simulink model "plant_control"  (R2023a)
settings: Solver=VariableStepAuto  StartTime=0.0  StopTime=10.0  RelTol=1e-3
settings Model: Creator=timme  LastModifiedBy=timme

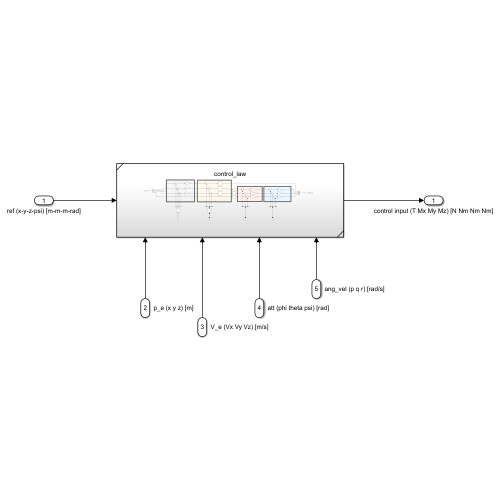
[thumbnail: Simulink's stored preview of the top-level diagram]
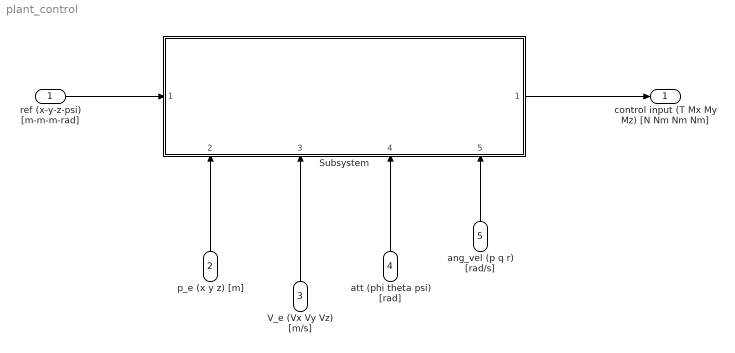
== system plant_control ==
  ref (x-y-z-psi) [m-m-m-rad] : Inport
  p_e (x y z) [m] : Inport  Port=2
  V_e (Vx Vy Vz) [m/s] : Inport  Port=3
  att (phi theta psi) [rad] : Inport  Port=4
  ang_vel (p q r) [rad/s] : Inport  Port=5
  Subsystem : Subsystem  ReferencedSubsystem=control_law
      settings: PortSchema="{\"entries\":[{\"content\":{\"sides\":[{\"content\":{\"connectorIds\":[\"In1\"]},\"type\":\"ConnectorPlacement.EquallySpacedRectSide\",\"uuid\":\"f752c7f8-b83e-4308-8655-52e5c72cb701\"},{\"content\":{\"connectorIds\":[\"Out1\"],\"side\":\"RIGHT\"},\"type\":\"ConnectorPlacement.EquallySpacedRectSide\",\"uuid\":\"74a5b19f-ee33-48e3-9b00-74ec74f49d4f\"},{\"content\":{\"side\":\"TOP\"},\"type\":\"ConnectorPlacement.EquallySpacedRectSide\",\"uuid\":\"54706187-071e-4a9a-98a6-285fd5b3a59a\"},{\"content\":{\"connectorIds\":[\"In2\",\"In3\",\"In4\",\"In5\"],\"side\":\"BOTTOM\"},\"type\":\"ConnectorPlacement.EquallySpacedRectSide\",\"uuid\":\"8e8e1002-9a2b-4fe1-9d78-42937cc6c4a1\"}]},\"type\":\"ConnectorPlacement.EquallySpacedConnector\",\"uuid\":\"c835d8d2-202e-4d2a-8f1b-a8986a5bc5c3\"}],\"packageUris\":[\"http://schema.mathworks.com/mf0/Connector/R2020b\"],\"version\":\"1.0\"}"
  control input (T Mx My Mz) [N Nm Nm Nm] : Outport
  wires:
  ref (x-y-z-psi) [m-m-m-rad]/1 -> Subsystem/1
  p_e (x y z) [m]/1 -> Subsystem/2
  V_e (Vx Vy Vz) [m/s]/1 -> Subsystem/3
  att (phi theta psi) [rad]/1 -> Subsystem/4
  ang_vel (p q r) [rad/s]/1 -> Subsystem/5
  Subsystem/1 -> control input (T Mx My Mz) [N Nm Nm Nm]/1
